simulink model "bd_par_auto2"  (Simulink 4.1.1)
settings: Solver=ode1  SolverMode=SingleTasking  StartTime=0.0  StopTime=max(cyc_mph(:,1))  FixedStep=1  MaxStep=1  RelTol=1e-3  AbsTol=1e-3
undefined symbols (not defined in the file): air_cp, amb_tmp, cs_charge_deplete_bool, cs_charge_trq, cs_electric_decel_spd, cs_electric_launch_spd_hi, cs_electric_launch_spd_lo, cs_hi_soc, cs_lo_soc, cs_min_trq_frac, cs_off_trq_frac, cyc_avg_time, cyc_cargo_mass, cyc_elevation_init, cyc_filter_bool, cyc_grade, cyc_mph, enable_stop, ess_cap_scale, ess_coulombic_eff, ess_init_soc, ess_max_ah_cap, ess_max_volts, ess_min_volts, ess_mod_airflow, ess_mod_cp, ess_mod_init_tmp, ess_module_mass, ess_module_num, ess_on, ess_res_scale_coef, ess_res_scale_fun, ess_set_tmp, ess_th_calc, ess_th_res_off, ess_th_res_on, ess_tmp, ess_voc, ex_calc, fc_ct_trq, fc_emis, fc_inertia, fc_map_spd, fc_max_trq, fc_on, fc_spd_scale, fc_trq_scale, fc_tstat, fd_inertia, fd_loss, fd_ratio, gb_dnshift_load, gb_dnshift_spd, gb_gears_num, gb_inertia, gb_num_init, gb_ratio, gb_shift_delay, gb_spd_scale, gb_trq_scale ... (+56)
libraries: lib_wheel2 x12, lib_accessory2 x3, lib_etc x2, lib_drive_cycle2 x1, lib_interactive x1, lib_drive_cycle x1, lib_exhaust x1, lib_fuel_converter3 x1
(part 11 of 18)

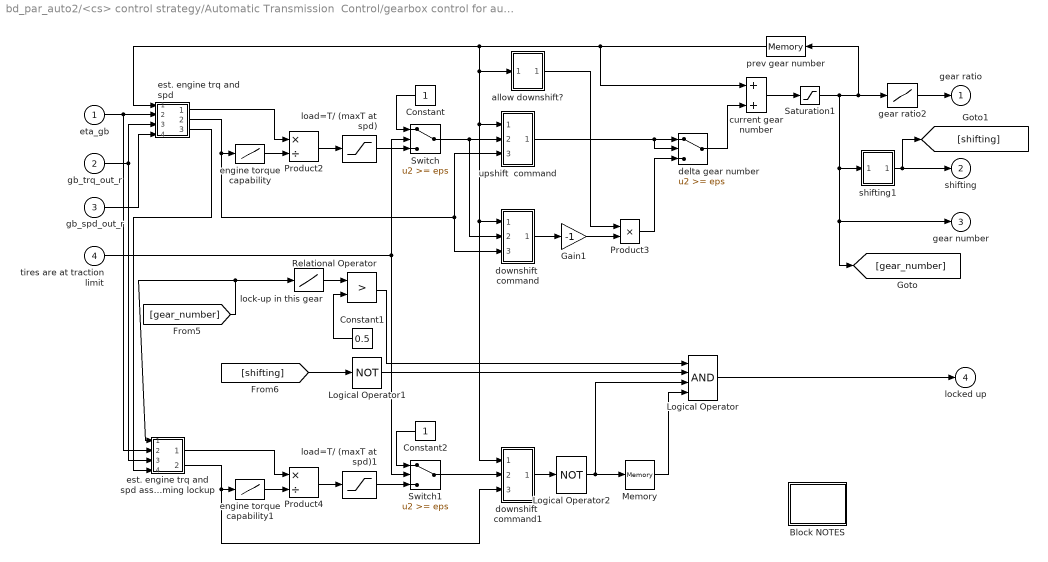
== system bd_par_auto2/<cs> control strategy/Automatic Transmission  Control/gearbox control for automatic transmission/gearbox control for use w/ AT ==
  eta_gb : Inport  Port=1  LatchInput=off
  gb_trq_out_r : Inport  Port=2  LatchInput=off
  gb_spd_out_r : Inport  Port=3  LatchInput=off
  tires are at traction limit : Inport  Port=4  LatchInput=off
  Block NOTES : Subsystem
      settings: RTWFcnNameOpts=Auto  RTWFileNameOpts=Auto
      mask Display: disp('Block\nNOTES')
  Constant : Constant  Orientation=left  Value=1
  Constant1 : Constant  Orientation=left  Value=0.5
  Constant2 : Constant  Orientation=left  Value=1
  Gain1 : Gain  Gain=-1  Multiplication=Element-wise(K.*u)  SaturateOnIntegerOverflow=on
  Logical Operator : Logic  Operator=AND  Inputs=4
  Logical Operator1 : Logic  Operator=NOT  Inputs=1
  Logical Operator2 : Logic  Operator=NOT  Inputs=1
  Memory : Memory  X0=0  InheritSampleTime=off
      settings: RTWStateStorageClass=Auto
  Product2 : Product  Inputs=*/  Multiplication=Element-wise(.*)  SaturateOnIntegerOverflow=on
  Product3 : Product  Inputs=2  Multiplication=Element-wise(.*)  SaturateOnIntegerOverflow=on
  Product4 : Product  Inputs=*/  Multiplication=Element-wise(.*)  SaturateOnIntegerOverflow=on
  Relational Operator : RelationalOperator  Operator=>
  Saturation1 : Saturate  UpperLimit=gb_gears_num  LowerLimit=1  LinearizeAsGain=on
  Switch : Switch  Threshold=eps
  Switch1 : Switch  Threshold=eps
  allow downshift? : Subsystem
      settings: RTWFcnNameOpts=Auto  RTWFileNameOpts=Auto
  current gear number : Sum  Inputs=++  SaturateOnIntegerOverflow=on
  delta gear number : Switch  Threshold=eps
  downshift  command : Subsystem
      settings: RTWFcnNameOpts=Auto  RTWFileNameOpts=Auto
  downshift  command1 : Subsystem
      settings: RTWFcnNameOpts=Auto  RTWFileNameOpts=Auto
  engine torque capability : Lookup  InputValues=fc_map_spd*fc_spd_scale  OutputValues=fc_max_trq*fc_trq_scale+eps
  engine torque capability1 : Lookup  InputValues=fc_map_spd*fc_spd_scale  OutputValues=fc_max_trq*fc_trq_scale+eps
  est. engine trq and spd : Subsystem
      settings: RTWFcnNameOpts=Auto  RTWFileNameOpts=Auto
  est. engine trq and spd assuming lockup : Subsystem
      settings: RTWFcnNameOpts=Auto  RTWFileNameOpts=Auto
  gear ratio2 : Lookup  InputValues=[1:length(gb_ratio)]  OutputValues=gb_ratio
  load=T/ (maxT at spd) : Saturate  UpperLimit=1  LowerLimit=-1  LinearizeAsGain=on
  load=T/ (maxT at spd)1 : Saturate  UpperLimit=1  LowerLimit=-1  LinearizeAsGain=on
  lock-up in this gear : Lookup  InputValues=[1:length(htc_lockup)]  OutputValues=htc_lockup
  prev gear number : Memory  Orientation=left  X0=gb_num_init  InheritSampleTime=off
      settings: RTWStateStorageClass=Auto
  shifting1 : Subsystem
      settings: RTWFcnNameOpts=Auto  RTWFileNameOpts=Auto
  upshift  command : Subsystem
      settings: RTWFcnNameOpts=Auto  RTWFileNameOpts=Auto
  gear ratio : Outport  Port=1  InitialOutput=0
  shifting : Outport  Port=2  InitialOutput=0
  gear number : Outport  Port=3  InitialOutput=0
  locked up : Outport  Port=4  InitialOutput=0
  wires:
  [gear_number] -> est. engine trq and spd assuming lockup/1(new gear number), lock-up in this gear/1
  [shifting] -> Logical Operator1/1
  lock-up in this gear/1 -> Relational Operator/1
  Constant1/1 -> Relational Operator/2
  shifting1/1(out_1) -> shifting/1, [shifting]
  downshift  command1/1(command) -> Logical Operator2/1
  load=T/ (maxT at spd)1/1 -> Switch1/3
  Memory/1 -> Logical Operator/4
  Switch1/1 -> downshift  command1/2(engine load)
  Logical Operator/1 -> locked up/1
  Gain1/1 -> Product3/2
  upshift  command/1(command) -> delta gear number/1, delta gear number/2
  Switch/1 -> upshift  command/2(engine load), downshift  command/2(engine load)
  Logical Operator2/1 -> Memory/1, Logical Operator/3
  est. engine trq and spd assuming lockup/2(est eng spd (rad/s)) -> downshift  command1/3(engine speed), engine torque capability1/1
  est. engine trq and spd/3(gb_spd_in_est (rad/s)) -> est. engine trq and spd assuming lockup/4(gb_spd_in_est)
  tires are at traction limit/1 -> Switch/2, Switch1/2
  gb_trq_out_r/1 -> est. engine trq and spd assuming lockup/3(gb_trq_out_r), est. engine trq and spd/3(gb_trq_out_r)
  eta_gb/1 -> est. engine trq and spd assuming lockup/2(" prev eta_gb"), est. engine trq and spd/2(" prev eta_gb")
  est. engine trq and spd assuming lockup/1(est eng trq (Nm)) -> Product4/1
  engine torque capability1/1 -> Product4/2
  Product4/1 -> load=T/ (maxT at spd)1/1
  Constant2/1 -> Switch1/1
  Relational Operator/1 -> Logical Operator/1
  Logical Operator1/1 -> Logical Operator/2
  downshift  command/1(command) -> Gain1/1
  load=T/ (maxT at spd)/1 -> Switch/3
  est. engine trq and spd/1(est eng trq (Nm)) -> Product2/1
  engine torque capability/1 -> Product2/2
  current gear number/1 -> Saturation1/1
  Product3/1 -> delta gear number/3
  allow downshift?/1(allow shift) -> Product3/1
  delta gear number/1 -> current gear number/2
  Product2/1 -> load=T/ (maxT at spd)/1
  Constant/1 -> Switch/1
  Saturation1/1 -> shifting1/1(gear number), gear number/1, [gear_number], prev gear number/1, gear ratio2/1
  prev gear number/1 -> est. engine trq and spd/1(prev gear number), allow downshift?/1(prev gearnum), downshift  command1/1(prev gear number), downshift  command/1(prev gear number), upshift  command/1(prev gear number), current gear number/1
  gear ratio2/1 -> gear ratio/1
  gb_spd_out_r/1 -> est. engine trq and spd/4(gb_spd_out_r)
  est. engine trq and spd/2(est eng spd (rad/s)) -> engine torque capability/1, upshift  command/3(engine speed), downshift  command/3(engine speed)

== system bd_par_auto2/<cs> control strategy/Clutch Control/Clutch Control/parallel clutch control ==
  shifting : Inport  Port=1  LatchInput=off
  gb_trq_in_r : Inport  Port=2  LatchInput=off
  gb_spd_in_r : Inport  Port=3  LatchInput=off
  engine on : Inport  Port=4  LatchInput=off
  Block NOTES : Subsystem
      settings: RTWFcnNameOpts=Auto  RTWFileNameOpts=Auto
      mask Display: disp('Block\nNOTES')
  Constant : Constant  Value=1e-3
  Constant1 : Constant  Value=vc_clutch_bool
  Constant2 : Constant  Value=vc_idle_spd
  Constant3 : Constant  Value=1e-3
  Constant4 : Constant  Value=vc_launch_spd
  Constant5 : Constant  Orientation=left  Value=2.5
  Constant6 : Constant  Orientation=left  Value=1
  Fcn: 1 if clutch disengaged 2 if clutch slipping 3 if clutch engaged : Fcn  Expr=u[1]+2*u[2]*(1-u[1])*(1-u[3])+3*u[3]*(1-u[1])
  Logical Operator : Logic  Operator=AND  Inputs=2
  Logical Operator1 : Logic  Operator=OR  Inputs=2
  Memory : Memory  Orientation=left  X0=1+(2*(cyc_mph(1,2)>0))  InheritSampleTime=off
      settings: RTWStateStorageClass=Auto
  Mux : Mux  Inputs=3
      settings: DisplayOption=none
  Relational Operator : RelationalOperator  Operator=<=
  Relational Operator1 : RelationalOperator  Operator=<
  Relational Operator2 : RelationalOperator  Operator=>
  Relational Operator3 : RelationalOperator  Operator=<
  Switch : Switch  Threshold=eps
  clutch disengaged : Logic  Operator=OR  Inputs=2
  clutch engaged : Logic  Operator=NOR  Inputs=2
  clutch slipping : Logic  Operator=AND  Inputs=3
  clutch was NOT fully engaged during last time step : RelationalOperator  Orientation=left  Operator=<
  gearbox speed estimator : Subsystem
      settings: RTWFcnNameOpts=Auto  RTWFileNameOpts=Auto
  clutch state : Outport  Port=1
  wires:
  Switch/1 -> Memory/1, clutch state/1
  Fcn: 1 if clutch disengaged 2 if clutch slipping 3 if clutch engaged/1 -> Switch/1
  gearbox speed estimator/1(Out1) -> Relational Operator3/1, Relational Operator1/1
  gb_spd_in_r/1 -> gearbox speed estimator/1(gb_spd_in_r if no gear change)
  engine on/1 -> Switch/2
  Relational Operator1/1 -> Logical Operator1/2
  Constant2/1 -> Relational Operator1/2
  Mux/1 -> Fcn: 1 if clutch disengaged 2 if clutch slipping 3 if clutch engaged/1
  clutch engaged/1 -> Mux/3
  clutch disengaged/1 -> clutch engaged/1, Mux/1
  Constant3/1 -> Relational Operator2/2
  Relational Operator2/1 -> clutch slipping/1
  clutch slipping/1 -> clutch engaged/2, Mux/2
  Constant4/1 -> Relational Operator3/2
  Relational Operator3/1 -> clutch slipping/2
  Memory/1 -> clutch was NOT fully engaged during last time step/1
  Constant5/1 -> clutch was NOT fully engaged during last time step/2
  clutch was NOT fully engaged during last time step/1 -> clutch slipping/3
  Constant1/1 -> Logical Operator1/1
  Constant/1 -> Relational Operator/2
  Relational Operator/1 -> Logical Operator/1
  Logical Operator1/1 -> Logical Operator/2
  gb_trq_in_r/1 -> Relational Operator2/1, Relational Operator/1
  Logical Operator/1 -> clutch disengaged/2
  shifting/1 -> clutch disengaged/1
  Constant6/1 -> Switch/3

== system bd_par_auto2/<cs> control strategy/Clutch Control/Clutch Control/repeated cycle:  speed required at end of NEXT step ==
  Clock : Clock
      settings: DisplayTime=off  Decimation=10
  Fcn1 : Fcn  Expr=rem(u[1],period)
  Look-Up Table : Lookup  InputValues=t  OutputValues=y
  Memory : Memory  X0=-0.1  InheritSampleTime=off
      settings: RTWStateStorageClass=Auto
  Sum : Sum  Inputs=+-  SaturateOnIntegerOverflow=on
  Sum1 : Sum  Inputs=++  SaturateOnIntegerOverflow=on
  out_1 : Outport  Port=1  InitialOutput=0
  wires:
  Clock/1 -> Sum/1, Memory/1, Fcn1/1
  Memory/1 -> Sum/2
  Sum/1 -> Sum1/2
  Fcn1/1 -> Sum1/1
  Look-Up Table/1 -> out_1/1
  Sum1/1 -> Look-Up Table/1

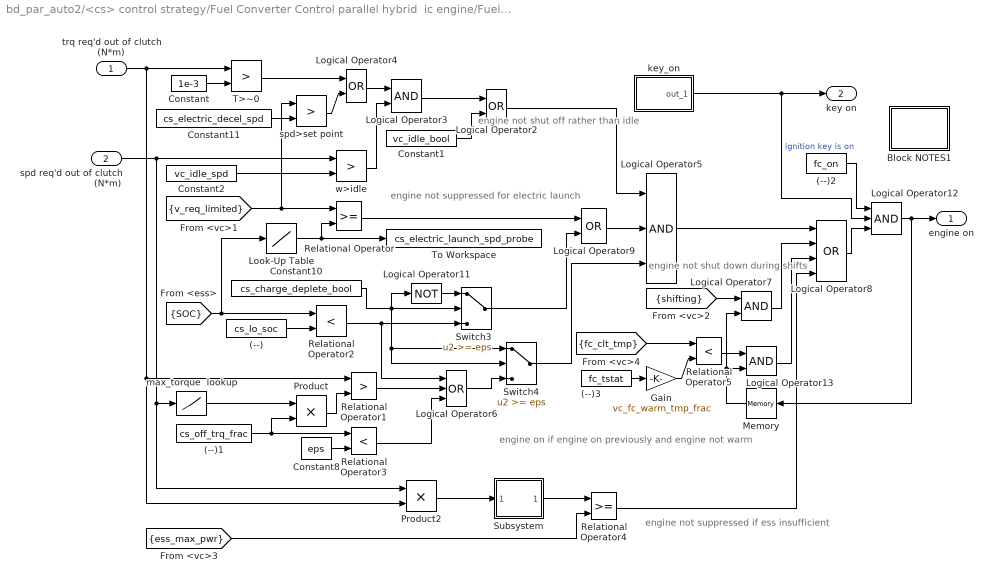
== system bd_par_auto2/<cs> control strategy/Fuel Converter Control parallel hybrid  ic engine/Fuel Converter Control/engine on (parallel hybrid) ==
  note: engine not shut
      | down during shifts
  note: engine on if engine on
      | previously and engine
      | not warm
  note: engine not shut off
      |  rather than idle
  note: engine not
      | suppressed for
      | electric launch
  note: engine not suppressed if
      | ess insufficient
  trq req'd out of clutch (N*m) : Inport  Port=1  LatchInput=off
  spd req'd out of clutch (N*m) : Inport  Port=2  LatchInput=off
  (--) : Constant  Value=cs_lo_soc
  (--)1 : Constant  Value=cs_off_trq_frac
  (--)2 : Constant  Value=fc_on
  (--)3 : Constant  Value=fc_tstat
  Block NOTES1 : Subsystem
      settings: RTWFcnNameOpts=Auto  RTWFileNameOpts=Auto
      mask Display: disp('Block\nNOTES')
  Constant : Constant  Value=1e-3
  Constant1 : Constant  Value=vc_idle_bool
  Constant10 : Constant  Value=cs_charge_deplete_bool
  Constant11 : Constant  Value=cs_electric_decel_spd
  Constant2 : Constant  Value=vc_idle_spd
  Constant8 : Constant  Value=eps
  Gain : Gain  Gain=vc_fc_warm_tmp_frac  Multiplication=Element-wise(K.*u)  SaturateOnIntegerOverflow=on
  Logical Operator11 : Logic  Operator=NOT  Inputs=1
  Logical Operator12 : Logic  Operator=AND  Inputs=3
  Logical Operator13 : Logic  Operator=AND  Inputs=2
  Logical Operator2 : Logic  Operator=OR  Inputs=2
  Logical Operator3 : Logic  Operator=AND  Inputs=2
  Logical Operator4 : Logic  Operator=OR  Inputs=2
  Logical Operator5 : Logic  Operator=AND  Inputs=3
  Logical Operator6 : Logic  Operator=OR  Inputs=3
  Logical Operator7 : Logic  Operator=AND  Inputs=2
  Logical Operator8 : Logic  Operator=OR  Inputs=4
  Logical Operator9 : Logic  Operator=OR  Inputs=2
  Look-Up Table : Lookup  InputValues=[cs_lo_soc cs_hi_soc cs_hi_soc+eps]  OutputValues=[cs_electric_launch_spd_lo cs_electric_launch_spd_hi cs_electric_launch_spd_hi]
  Memory : Memory  Orientation=left  X0=cyc_mph(1,2)>0  InheritSampleTime=off
      settings: RTWStateStorageClass=Auto
  Product : Product  Inputs=2  Multiplication=Element-wise(.*)  SaturateOnIntegerOverflow=on
  Product2 : Product  Inputs=2  Multiplication=Element-wise(.*)  SaturateOnIntegerOverflow=on
  Relational Operator : RelationalOperator  Operator=>=
  Relational Operator1 : RelationalOperator  Operator=>
  Relational Operator2 : RelationalOperator  Operator=<
  Relational Operator3 : RelationalOperator  Operator=<
  Relational Operator4 : RelationalOperator  Operator=>=
  Relational Operator5 : RelationalOperator  Operator=<
  Subsystem : Subsystem  mask(Running Average){n=3}
      mask prompts: n "Averaging Time Steps (#)"
      mask help: Running Average
      settings: RTWFcnNameOpts=Auto  RTWFileNameOpts=Auto
      mask Help: Output is the average of the last (Averaging Time) seconds of input.
      mask Display: disp('Running\nAverage')
  Switch3 : Switch  Threshold=eps
  Switch4 : Switch  Threshold=eps
  T>~0 : RelationalOperator  Operator=>
  To Workspace : ToWorkspace  VariableName=cs_electric_launch_spd_probe  SampleTime=-1  SaveFormat=Array
  key_on : Subsystem  mask(Repeating table){@1=vc_key_on(:,1), @2=vc_key_on(:,2)}
      mask prompts: @1 "Time values:"; @2 "Output values:"
      mask help:
      | Repeating table.
      | Enter values of time and output for first cycle.
      mask init:
      | period = max(@1); t = @1; y = @2;
      settings: RTWFcnNameOpts=Auto  RTWFileNameOpts=Auto
      mask Help: Repeats cycle given in table. Time values should be monotonically increasing.
  max_torque  lookup : Lookup  InputValues=fc_map_spd*fc_spd_scale  OutputValues=fc_max_trq*fc_trq_scale
  spd>set point : RelationalOperator  Operator=>
  w>idle : RelationalOperator  Operator=>
  engine on : Outport  Port=1
  key on : Outport  Port=2
  wires:
  Subsystem/1(out_1) -> Relational Operator4/1
  [v_req_limited] -> spd>set point/1, Relational Operator/1
  Logical Operator4/1 -> Logical Operator3/1
  T>~0/1 -> Logical Operator4/1
  spd>set point/1 -> Logical Operator4/2
  Constant11/1 -> spd>set point/2
  Relational Operator4/1 -> Logical Operator8/4
  Product2/1 -> Subsystem/1(in_1)
  [ess_max_pwr] -> Relational Operator4/2
  (--)/1 -> Relational Operator2/2
  [SOC] -> Look-Up Table/1, Relational Operator2/1
  Logical Operator11/1 -> Switch3/1
  Relational Operator2/1 -> Logical Operator6/1, Switch3/3
  Constant10/1 -> Logical Operator11/1, Switch3/2, Switch4/2, Switch4/1
  Look-Up Table/1 -> To Workspace/1, Relational Operator/2
  Relational Operator/1 -> Logical Operator9/1
  Switch4/1 -> Logical Operator5/3
  Logical Operator9/1 -> Logical Operator5/2
  Logical Operator2/1 -> Logical Operator5/1
  key_on/1(out_1) -> Logical Operator12/2, key on/1  "ignition key is on"
  Logical Operator8/1 -> Logical Operator12/3
  (--)3/1 -> Gain/1
  Gain/1 -> Relational Operator5/2
  Logical Operator13/1 -> Logical Operator8/3
  [fc_clt_tmp] -> Relational Operator5/1
  Relational Operator5/1 -> Logical Operator13/1
  Memory/1 -> Logical Operator13/2, Logical Operator7/2
  Relational Operator1/1 -> Logical Operator6/2
  Logical Operator5/1 -> Logical Operator8/1
  spd req'd out of clutch (N*m)/1 -> w>idle/1, max_torque  lookup/1, Product2/1
  w>idle/1 -> Logical Operator3/2
  Logical Operator3/1 -> Logical Operator2/1
  Constant1/1 -> Logical Operator2/2
  trq req'd out of clutch (N*m)/1 -> Relational Operator1/1, Product2/2, T>~0/1
  Logical Operator7/1 -> Logical Operator8/2
  [shifting] -> Logical Operator7/1
  Constant/1 -> T>~0/2
  Constant2/1 -> w>idle/2
  Switch3/1 -> Logical Operator9/2
  Logical Operator6/1 -> Switch4/3
  Relational Operator3/1 -> Logical Operator6/3
  Constant8/1 -> Relational Operator3/2
  (--)1/1 -> Relational Operator3/1, Product/2
  Product/1 -> Relational Operator1/2
  max_torque  lookup/1 -> Product/1
  (--)2/1 -> Logical Operator12/1
  Logical Operator12/1 -> engine on/1, Memory/1

== system bd_par_auto2/<cs> control strategy/Hybrid  Engine Torque Modification Strategy/parallel auto hybrid torque control/chg trq req'd (Nm) ==
  SOC : Inport  Port=1  LatchInput=off
  Constant : Constant  Value=cs_charge_trq*fc_trq_scale
  Constant1 : Constant  Value=ess_on
  Goal : Constant  Value=(cs_lo_soc+cs_hi_soc)/2
  Product : Product  Inputs=2  Multiplication=Element-wise(.*)  SaturateOnIntegerOverflow=on
  Product1 : Product  Inputs=*/  Multiplication=Element-wise(.*)  SaturateOnIntegerOverflow=on
  Range : Constant  Value=(cs_hi_soc-cs_lo_soc)/2
  Saturation : Saturate  UpperLimit=inf  LowerLimit=-inf  LinearizeAsGain=on
  Sum : Sum  Inputs=-+  SaturateOnIntegerOverflow=on
  Switch : Switch  Threshold=eps
  add'l trq req'd (Nm) : Outport  Port=1
  wires:
  Constant1/1 -> Switch/3, Switch/2
  Switch/1 -> add'l trq req'd (Nm)/1
  Saturation/1 -> Switch/1
  Goal/1 -> Sum/2
  Range/1 -> Product1/2
  Sum/1 -> Product1/1
  Product1/1 -> Product/2
  Constant/1 -> Product/1
  Product/1 -> Saturation/1
  SOC/1 -> Sum/1

== system bd_par_auto2/<cs> control strategy/Hybrid  Engine Torque Modification Strategy/parallel auto hybrid torque control/minimum trq (Nm) ==
  "spd req'd in (N*m, rad/s)" : Inport  Port=1  LatchInput=off
  SOC : Inport  Port=2  LatchInput=off
  (--) : Constant  Value=cs_lo_soc
  Constant : Constant  Value=0
  Gain : Gain  Gain=cs_min_trq_frac  Multiplication=Element-wise(K.*u)  SaturateOnIntegerOverflow=on
  Relational Operator2 : RelationalOperator  Operator=<
  Switch : Switch  Threshold=eps
  max_torque lookup : Lookup  InputValues=fc_map_spd  OutputValues=fc_max_trq*fc_trq_scale
  minimum trq (N*m) : Outport  Port=1
  wires:
  Gain/1 -> Switch/1
  max_torque lookup/1 -> Gain/1
  "spd req'd in (N*m, rad/s)"/1 -> max_torque lookup/1
  Constant/1 -> Switch/3
  Switch/1 -> minimum trq (N*m)/1
  Relational Operator2/1 -> Switch/2
  (--)/1 -> Relational Operator2/2
  SOC/1 -> Relational Operator2/1

== system bd_par_auto2/ACC MECH <accm>/mechanical accessory model and interface/Mechanical Accessory model/Block NOTES ==
  note: In this model, only one speed is used to predict accessory
      | loading. The forward model is "dummied" out.
  note: A third input is given for accessory load speed. This is done so that
      | the accessory block can use fc_spd_est which is an estimated vehicle speed
      | (equal to fc_spd_out under normal circumstances).
      | Using fc_spd_est provides total compatibility with ADVISOR v3.2
  note: In terms of an interface, the model assumes belt-driven mechanical loads
      | that run off of a prime mover shaft (e.g., engine shaft)
      |
      | This model takes in requested driveline torque and speed requests and
      | augments torque due to belt driven accessories.
      |
      | The torque passed along down to the driveline is only torque to move the
      | vehicle.
  note: This is the mechanical auxiliary loads model.

== system bd_par_auto2/ACC MECH <accm>/mechanical accessory model and interface/Mechanical Accessory model/backward model ==
  note: Power, W, input to accessory
  note: T, Nm, shaft out
  note: T, Nm, driveline
  note: T, Nm, accessory
  note: w_apu, rad/s
  trq1 : Inport  Port=1  LatchInput=off
  spd_in : Inport  Port=2  LatchInput=off
  Product : Product  Inputs=**  Multiplication=Element-wise(.*)  SaturateOnIntegerOverflow=on
  Product1 : Product  Inputs=**  Multiplication=Element-wise(.*)  SaturateOnIntegerOverflow=on
  Sum : Sum  Inputs=|++  SaturateOnIntegerOverflow=on
  enhancedToWorkspace : Subsystem  TreatAsAtomicUnit=on  mask(enhancedToWorkspace){generalName=generalName, specificName=mech_pwr_r, logFlag=logFlag}
      mask prompts: generalName "General Name [char-evaluated]"; specificName "Specific Name [char-literal]"; logFlag "Enable flag (1=on,0=off)"
      mask help: A wrapper for the Simulink "To Workspace" block that allows you to evaluate the name of the variable to log to workspace. This is useful to avoid the double logging errors that occur when you pull in two library models that attempt to log to the same variable.
      mask init:
      | enhancedToWsMaker
      settings: CopyFcn=breakLinkCopyFcn  ParentCloseFcn=breakLinkParCloseFcn  RTWFcnNameOpts=Auto  RTWFileNameOpts=Auto
      mask Help:
      | <h2>Enhanced To Workspace Block</h2>
      | <h3>Parameters</h3>
      | <UL>
      | <li><b>General Name:</b> This is the more general name of the variable. Variables are saved to the workspace as <i>generalName_specificName</i>. Note that this is an evaluated variable. If you would like to type in the value directly, it must be surrounded with single quotes. Otherwise you can input the name of a variable containing a char string.</li>
      | <li><b>Specific Name:</b> This is the specific name of the variable. Note that this is input as a char literal (i.e., you don't need quotes).</li>
      | <li><b>Enable Flag:</b> This flag should have the value of 0 or 1. If 0, the variable will not be logged to the workspace. If 1, the variable will be logged. This is done so that variable logging can be turned off to improve speed.</li>
      | </ul>
      | <h3>Overview</h3>
      | <p>The enhanced to workspace block was put together to allow one to dynamically resolve variable names at run time in simulink. This is most powerful when used in conjunction with a masked subsystem to allow multiple instances of that masked subsytem to be used in the same model. The strategy is to set the generalName in the block mask which will allow the block to change the general name for all variable logging on the fly.
      | <h3>Helper Files</h3>
      | <p>Three m-files are required by the enhancedToWorkspace block. These files are located in the &lt; ADVISOR root &gt;/GUI directory :
      | <ul>
      | <li><i>enhancedToWsMaker.m</i> This file runs the mask initialization for the block</li>
      | <li><i>breakLinkCopyFcn.m</i> This file is used by the block callback when the simulink block is copied. It is necessary to break the link to the enhancedToWorkspace similar to the To Workspace block in order for it to be able to configure itself. (Try copying simulink's To Workspace block--it is impossible to make a link)</li>
      | <li><i>breakLinkParCloseFcn.m</i> This file is similar to the breakLinkCopyFcn and is used when a parent system is closed</li>
      | </ul>
      | <hr>
      | 
      | <p>Created 2003-Jan-21, Michael Patrick O'Keefe, NREL</p>
      | 
      | <!--
      | <VARDEF>
      | <H3>var_name</H3>
      | <UL>
      | <LI><B>data type</B> data type here</LI>
      | <LI><B>units</B> units here</LI>
      | <LI><B>vehicle type</B> vehicle type here</LI>
      | <LI><B>description</B> description here</LI>
      | </UL>
      | </VARDEF>
      | -->
      mask Display: disp([generalName,'_',specificName])
  enhancedToWorkspace1 : Subsystem  TreatAsAtomicUnit=on  mask(enhancedToWorkspace){generalName=generalName, specificName=mech_trq_r, logFlag=logFlag}
      mask prompts: generalName "General Name [char-evaluated]"; specificName "Specific Name [char-literal]"; logFlag "Enable flag (1=on,0=off)"
      mask help: A wrapper for the Simulink "To Workspace" block that allows you to evaluate the name of the variable to log to workspace. This is useful to avoid the double logging errors that occur when you pull in two library models that attempt to log to the same variable.
      mask init:
      | enhancedToWsMaker
      settings: CopyFcn=breakLinkCopyFcn  ParentCloseFcn=breakLinkParCloseFcn  RTWFcnNameOpts=Auto  RTWFileNameOpts=Auto
      mask Help:
      | <h2>Enhanced To Workspace Block</h2>
      | <h3>Parameters</h3>
      | <UL>
      | <li><b>General Name:</b> This is the more general name of the variable. Variables are saved to the workspace as <i>generalName_specificName</i>. Note that this is an evaluated variable. If you would like to type in the value directly, it must be surrounded with single quotes. Otherwise you can input the name of a variable containing a char string.</li>
      | <li><b>Specific Name:</b> This is the specific name of the variable. Note that this is input as a char literal (i.e., you don't need quotes).</li>
      | <li><b>Enable Flag:</b> This flag should have the value of 0 or 1. If 0, the variable will not be logged to the workspace. If 1, the variable will be logged. This is done so that variable logging can be turned off to improve speed.</li>
      | </ul>
      | <h3>Overview</h3>
      | <p>The enhanced to workspace block was put together to allow one to dynamically resolve variable names at run time in simulink. This is most powerful when used in conjunction with a masked subsystem to allow multiple instances of that masked subsytem to be used in the same model. The strategy is to set the generalName in the block mask which will allow the block to change the general name for all variable logging on the fly.
      | <h3>Helper Files</h3>
      | <p>Three m-files are required by the enhancedToWorkspace block. These files are located in the &lt; ADVISOR root &gt;/GUI directory :
      | <ul>
      | <li><i>enhancedToWsMaker.m</i> This file runs the mask initialization for the block</li>
      | <li><i>breakLinkCopyFcn.m</i> This file is used by the block callback when the simulink block is copied. It is necessary to break the link to the enhancedToWorkspace similar to the To Workspace block in order for it to be able to configure itself. (Try copying simulink's To Workspace block--it is impossible to make a link)</li>
      | <li><i>breakLinkParCloseFcn.m</i> This file is similar to the breakLinkCopyFcn and is used when a parent system is closed</li>
      | </ul>
      | <hr>
      | 
      | <p>Created 2003-Jan-21, Michael Patrick O'Keefe, NREL</p>
      | 
      | <!--
      | <VARDEF>
      | <H3>var_name</H3>
      | <UL>
      | <LI><B>data type</B> data type here</LI>
      | <LI><B>units</B> units here</LI>
      | <LI><B>vehicle type</B> vehicle type here</LI>
      | <LI><B>description</B> description here</LI>
      | </UL>
      | </VARDEF>
      | -->
      mask Display: disp([generalName,'_',specificName])
  mechanical accessories (Nm) : Subsystem  BlockChoice=Mechanical Accessories: Const Mech Var Elect
      settings: AttributesFormatString=%<BlockChoice>  MemberBlocks=Mechanical Accessories: Const Mech Var Elect,Mechanical Accessories: Constant Mechanical & Electrical,Mechanical Accessories: Speed Dependant and Variable Electrical,Saber Dual Voltage Cosim,Saber Single Voltage Cosim,SindaTransAC  RTWFcnNameOpts=Auto  RTWFileNameOpts=Auto
      settings: TemplateBlock=|
      | lib_accessory2/ACC MECH
      | models/mechanical accessories (Nm)
      mask Display: image(imread('bdi_acc_pic_cs.bmp'))
  trq2 : Outport  Port=1
  tag scope: acc_mech_pwr_r=scoped, acc_mech_trq_r=scoped
  wires:
  [acc_on] -> Product1/2
  [acc_on] -> Product/1
  mechanical accessories (Nm)/2(P_mech_acc) -> Product1/1
  Product1/1 -> enhancedToWorkspace/1(In1), [acc_mech_pwr_r]
  mechanical accessories (Nm)/1(T_acc) -> Product/2
  Product/1 -> enhancedToWorkspace1/1(In1), [acc_mech_trq_r], Sum/2
  Sum/1 -> trq2/1
  trq1/1 -> Sum/1
  spd_in/1 -> mechanical accessories (Nm)/1(w_APU)

== system bd_par_auto2/ACC MECH <accm>/mechanical accessory model and interface/Mechanical Accessory model/f1 ==
  In1 : Inport  Port=1  LatchInput=off
  To Workspace : ToWorkspace  VariableName=accm_mech_pwr_a  SampleTime=-1  SaveFormat=Array
  wires:
  In1/1 -> To Workspace/1

== system bd_par_auto2/ACC MECH <accm>/mechanical accessory model and interface/Mechanical Accessory model/f2 ==
  In1 : Inport  Port=1  LatchInput=off
  To Workspace : ToWorkspace  VariableName=accm_mech_trq_a  SampleTime=-1  SaveFormat=Array
  wires:
  In1/1 -> To Workspace/1

== system bd_par_auto2/ACC MECH <accm>/mechanical accessory model and interface/Mechanical Accessory model/forward model ==
  note: pm trq a ==> prime mover (engine/fuel converter/input shaft driving accessories) torque achieved
      | acc spd ==> accessory reference shaft speed (may or may not be the same as the engine shaft speed
      | acc trq requested ==> accessory torque requested
  note: acc torque, Nm
  note: NOTES
  note: This simplistic model may not correctly account for accessory torque and/or power
      | when the upstream torque provider is torque or speed limited
  note: Power, W, input to accessory
  note: T, Nm, shaft out
  note: driveline and
      | acc torque, Nm
  note: T, Nm, accessory
  note: acc speed, rad/s
  trq_in : Inport  Port=1  LatchInput=off
  spd_in : Inport  Port=2  LatchInput=off
  acc_trq_req : Inport  Port=3  LatchInput=off
  Product1 : Product  Inputs=**  Multiplication=Element-wise(.*)  SaturateOnIntegerOverflow=on
  Sum : Sum  Inputs=|+-  SaturateOnIntegerOverflow=on
  trq_out : Outport  Port=1
  acc_mech_trq_a : Outport  Port=2
  acc_mech_pwr_a : Outport  Port=3
  wires:
  [pm_trq_a] -> Sum/1
  acc_trq_req/1 -> [acc_trq_r]
  trq_in/1 -> [pm_trq_a]
  [acc_spd] -> Product1/2
  [acc_trq_r] -> Product1/1, Sum/2, acc_mech_trq_a/1
  Product1/1 -> acc_mech_pwr_a/1
  Sum/1 -> trq_out/1
  spd_in/1 -> [acc_spd]

== system bd_par_auto2/ACC MECH <accm>/mechanical accessory model and interface/signal annotator/enhancedToWorkspace ==
  In1 : Inport  Port=1  LatchInput=off
  To Workspace : ToWorkspace  VariableName=accm_pre_acc_spd_out_r  SampleTime=-1  SaveFormat=Array
  wires:
  In1/1 -> To Workspace/1

== system bd_par_auto2/ACC MECH <accm>/mechanical accessory model and interface/signal annotator/enhancedToWorkspace1 ==
  In1 : Inport  Port=1  LatchInput=off
  To Workspace : ToWorkspace  VariableName=accm_pre_acc_trq_out_r  SampleTime=-1  SaveFormat=Array
  wires:
  In1/1 -> To Workspace/1

== system bd_par_auto2/clutch <cl>/clutch model and interface/clutch model/Adjust for Possible Launch Speed Request ==
  note: If the clutch is disengaged, under certain
      | circumstances, we will want to request that
      | the input speed to the clutch be ramped up to a
      | given launch speed (decided by the controller)
      | so that the clutch can subsequently slip and
      | engage with a more realistic speed matching
  Input Speed Request : Inport  Port=1  LatchInput=off
  Constant6 : Constant  Value=1
  Logical Operator : Logic  Operator=AND  Inputs=2
  Switch4 : Switch  Threshold=0.5
  clutch disengaged : RelationalOperator  Operator===
  Input Speed Request Adjusted for Launch Speed : Outport  Port=1
  wires:
  Logical Operator/1 -> Switch4/2
  clutch disengaged/1 -> Logical Operator/2
  [launch_flag] -> Logical Operator/1
  Constant6/1 -> clutch disengaged/2
  [clutch_state] -> clutch disengaged/1
  Input Speed Request/1 -> Switch4/3
  Switch4/1 -> Input Speed Request Adjusted for Launch Speed/1
  [launch_speed] -> Switch4/1

== system bd_par_auto2/clutch <cl>/clutch model and interface/clutch model/enhancedToWorkspace ==
  In1 : Inport  Port=1  LatchInput=off
  Terminator : Terminator
  wires:
  In1/1 -> Terminator/1

== system bd_par_auto2/clutch <cl>/clutch model and interface/clutch model/enhancedToWorkspace1 ==
  In1 : Inport  Port=1  LatchInput=off
  Terminator : Terminator
  wires:
  In1/1 -> Terminator/1

== system bd_par_auto2/clutch <cl>/clutch model and interface/clutch model/enhancedToWorkspace2 ==
  In1 : Inport  Port=1  LatchInput=off
  Terminator : Terminator
  wires:
  In1/1 -> Terminator/1

== system bd_par_auto2/clutch <cl>/clutch model and interface/clutch model/enhancedToWorkspace3 ==
  In1 : Inport  Port=1  LatchInput=off
  Terminator : Terminator
  wires:
  In1/1 -> Terminator/1

== system bd_par_auto2/clutch <cl>/clutch model and interface/clutch model/enhancedToWorkspace4 ==
  In1 : Inport  Port=1  LatchInput=off
  Terminator : Terminator
  wires:
  In1/1 -> Terminator/1

== system bd_par_auto2/clutch <cl>/clutch model and interface/clutch model/enhancedToWorkspace5 ==
  In1 : Inport  Port=1  LatchInput=off
  Terminator : Terminator
  wires:
  In1/1 -> Terminator/1

== system bd_par_auto2/clutch <cl>/clutch model and interface/clutch model/enhancedToWorkspace6 ==
  In1 : Inport  Port=1  LatchInput=off
  Terminator : Terminator
  wires:
  In1/1 -> Terminator/1

== system bd_par_auto2/clutch <cl>/clutch model and interface/clutch model/enhancedToWorkspace7 ==
  In1 : Inport  Port=1  LatchInput=off
  Terminator : Terminator
  wires:
  In1/1 -> Terminator/1

== system bd_par_auto2/clutch <cl>/clutch model and interface/clutch model/enhancedToWorkspace8 ==
  In1 : Inport  Port=1  LatchInput=off
  Terminator : Terminator
  wires:
  In1/1 -> Terminator/1

== system bd_par_auto2/clutch <cl>/clutch model and interface/clutch model/enhancedToWorkspace9 ==
  In1 : Inport  Port=1  LatchInput=off
  Terminator : Terminator
  wires:
  In1/1 -> Terminator/1

== system bd_par_auto2/clutch <cl>/clutch model and interface/clutch model/help ==

== system bd_par_auto2/drive cycle <cyc>/drive cycle model and interface/drive cycle model/Block NOTES ==
  note: This block determines the speed required of the vehicle.  If cyc_filter_bool
      | is true, a centered-in-time average of the trace, with backlash, is required of
      | the vehicle.  This may be useful to smooth out jumps in the trace.  Otherwise,
      | the trace, exactly as published, is required of the vehicle.
      | This block also determines the roadway grade of the cycle and the
      | elevation as a function of the distance travelelled

== system bd_par_auto2/drive cycle <cyc>/drive cycle model and interface/drive cycle model/distance travelled (m) ==
  Block NOTES : Subsystem
      settings: RTWFcnNameOpts=Auto  RTWFileNameOpts=Auto
      mask Display: disp('Block\nNOTES')
  Integrator : Integrator  ExternalReset=none  InitialConditionSource=internal  InitialCondition=0  LimitOutput=off  UpperSaturationLimit=inf  LowerSaturationLimit=-inf  ShowSaturationPort=off  ShowStatePort=off  AbsoluteTolerance=auto
  mph-->m/s : Gain  Gain=0.447  Multiplication=Element-wise(K.*u)  SaturateOnIntegerOverflow=on
  Out1 : Outport  Port=1  InitialOutput=0
  wires:
  mph-->m/s/1 -> Integrator/1
  [mpha] -> mph-->m/s/1
  Integrator/1 -> Out1/1

== system bd_par_auto2/drive cycle <cyc>/drive cycle model and interface/drive cycle model/enhancedToWorkspace ==
  In1 : Inport  Port=1  LatchInput=off
  To Workspace : ToWorkspace  VariableName=cyc_cargo_mass_vs_time  SampleTime=-1  SaveFormat=Array
  wires:
  In1/1 -> To Workspace/1

== system bd_par_auto2/drive cycle <cyc>/drive cycle model and interface/drive cycle model/repeated cycle grade vs. distance ==
  distance travelled (m) : Inport  Port=1  LatchInput=off
  Fcn1 : Fcn  Expr=rem(u[1],period)
  Look-Up Table : Lookup  InputValues=t  OutputValues=y
  out_1 : Outport  Port=1  InitialOutput=0
  wires:
  Look-Up Table/1 -> out_1/1
  Fcn1/1 -> Look-Up Table/1
  distance travelled (m)/1 -> Fcn1/1

== system bd_par_auto2/drive cycle <cyc>/drive cycle model and interface/drive cycle model/repeated cycle speed vs. time ==
  Clock : Clock
      settings: DisplayTime=off  Decimation=10
  Fcn1 : Fcn  Expr=rem(u[1],period)
  Look-Up Table : Lookup  InputValues=t  OutputValues=y
  out_1 : Outport  Port=1  InitialOutput=0
  wires:
  Look-Up Table/1 -> out_1/1
  Clock/1 -> Fcn1/1
  Fcn1/1 -> Look-Up Table/1

== system bd_par_auto2/drive cycle <cyc>/drive cycle model and interface/drive cycle model/super-smooth, no-lag trace ==
  Subsystem : Subsystem  mask(Running Average){@1=avgtime}
      mask prompts: @1 "Averaging Time (s)"
      mask help: Running Average
      mask init:
      | n=@1;
      settings: RTWFcnNameOpts=Auto  RTWFileNameOpts=Auto
      mask Help: Output is the average of the last (Averaging Time) seconds of input.
      mask Display: disp('Running\nAverage')
  repeated cycle : Subsystem
      settings: RTWFcnNameOpts=Auto  RTWFileNameOpts=Auto
  out_1 : Outport  Port=1  InitialOutput=0
  wires:
  repeated cycle/1(out_1) -> Subsystem/1(in_1)
  Subsystem/1(out_1) -> out_1/1
